simulink model "Task3"  (R2022b)
settings: Solver=VariableStepAuto  StartTime=0.0  StopTime=10.0  RelTol=1e-3
values from neighbouring files (symbols this model uses):
  A = [1 3 ... (first row only)    [Task_3.m]    (also in Task_5.m = [-1.460,0, 2.4276)
  B = [1 ... (first row only)    [Task_3.m]    (also in Task_5.m = [0.4182, 5.2026)
  K = linspace(0,2,1000)    [Task_1.m]    (also in Task_3.m = lqr(A_aug,B_aug,Q,R))
  r = 1.0    (= 1)    [Task_3.m]    (also in Task_5.m = [1,0;0,1;1,1;1,-1])
settings Model: Creator=geokr  LastModifiedBy=geokr

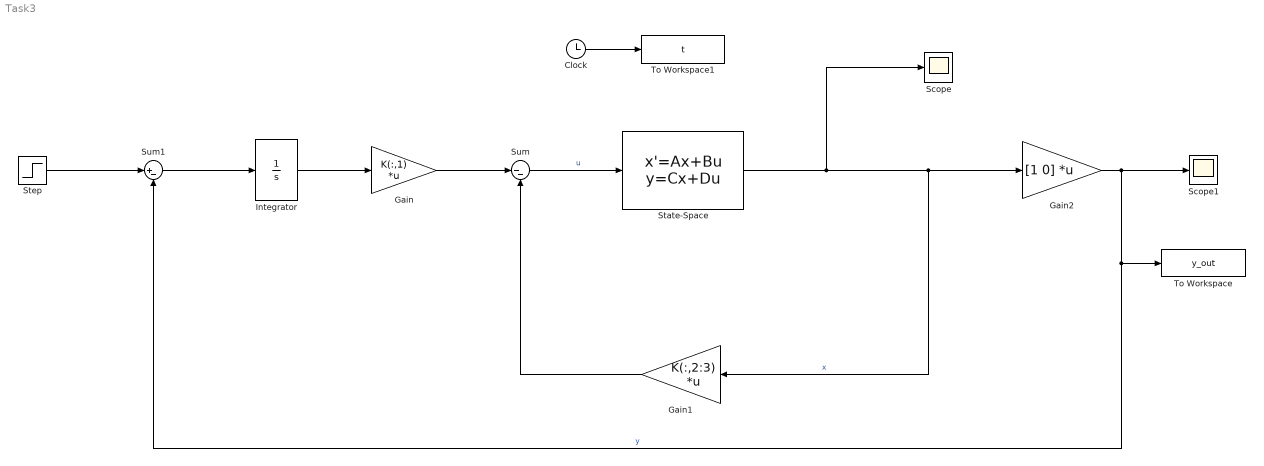
== system Task3 ==
  Clock : Clock
  Gain : Gain  Gain=K(:,1)  Multiplication=Matrix(K*u)
  Gain1 : Gain  Gain=K(:,2:3)  Multiplication=Matrix(K*u)
  Gain2 : Gain  Gain=[1 0]  Multiplication=Matrix(K*u)
  Integrator : Integrator
  Scope : Scope
  Scope1 : Scope
  State-Space : StateSpace  A=A  B=B  C=eye(2)  D=zeros(2,1)  InitialCondition=[0 0]  ParameterTunability=Unconstrained
  Step : Step  Time=0  After=r  SampleTime=0
  Sum : Sum  Inputs=|--
  Sum1 : Sum  Inputs=|+-
  To Workspace : ToWorkspace  VariableName=y_out  SampleTime=-1
  To Workspace1 : ToWorkspace  VariableName=t  SampleTime=-1
  wires:
  Gain1/1 -> Sum/2
  Sum/1 -> State-Space/1  "u"
  State-Space/1 -> Scope/1, Gain2/1, Gain1/1  "x"
  Gain2/1 -> To Workspace/1, Sum1/2, Scope1/1  "y"
  Step/1 -> Sum1/1
  Clock/1 -> To Workspace1/1
  Gain/1 -> Sum/1
  Integrator/1 -> Gain/1
  Sum1/1 -> Integrator/1
